simulink subsystem "omega_matrix"  (R2023b)
settings: Solver=VariableStepAuto  StartTime=0.0  StopTime=10.0  RelTol=1e-3
settings Model: Creator=pierb  LastModifiedBy=pierb

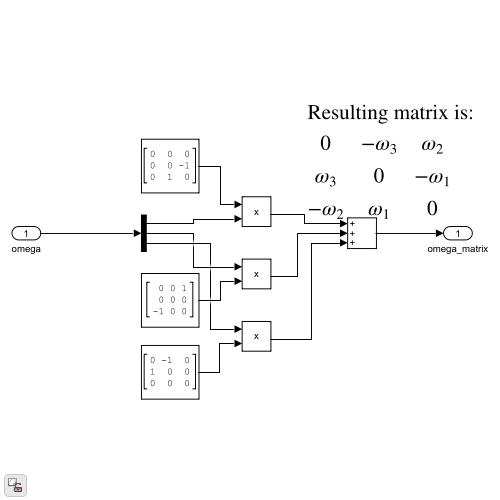
[thumbnail: Simulink's stored preview of the top-level diagram]
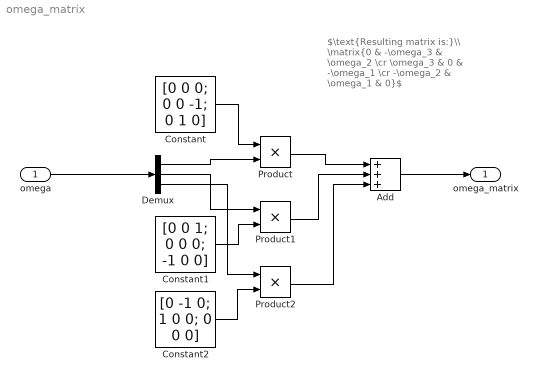
== system omega_matrix ==
  note: $\text{Resulting matrix is:}\\ \matrix{0 & -\omega_3 & \omega_2 \cr \omega_3 & 0 & -\omega_1 \cr -\omega_2 & \omega_1 & 0}$
  omega : Inport
  Add : Sum  Inputs=+++
  Constant : Constant  Value=[0 0 0; 0 0 -1; 0 1 0]
  Constant1 : Constant  Value=[0 0 1; 0 0 0; -1 0 0]
  Constant2 : Constant  Value=[0 -1 0; 1 0 0; 0 0 0]
  Demux : Demux  Outputs=3
  Product : Product
  Product1 : Product
  Product2 : Product
  omega_matrix : Outport
  wires:
  omega/1 -> Demux/1
  Constant/1 -> Product/1
  Demux/1 -> Product/2
  Demux/2 -> Product1/1
  Constant1/1 -> Product1/2
  Constant2/1 -> Product2/2
  Demux/3 -> Product2/1
  Product/1 -> Add/1
  Product1/1 -> Add/2
  Product2/1 -> Add/3
  Add/1 -> omega_matrix/1
